simulink model "Filter_main"  (R2023a)
settings: Solver=FixedStepDiscrete  StartTime=0.0  StopTime=2  FixedStep=Ts  RelTol=1e-3
InitFcn:
  | Ts=5e-6;
  | f=50;
  | w=2*pi*f;
libraries: spsThreePhaseSeriesRLCBranchLib x7, spsGroundLib x5, spsSeriesRLCBranchLib x3, spsThreePhaseVIMeasurementLib x3, powerlib_extras x2, spsRMSLib x2, spsTHDLib x2, spsThreePhaseParallelRLCLoadLib x2, spsThreePhaseHarmonicFilterLib x1, dspxfrm3 x1, spsPower3phInstantaneousLib x1, spsThreePhaseBreakerLib x1
settings Model: Creator=Aminsystem  LastModifiedBy=Aminsystem
settings DataIOCC: SaveOutput=off  SignalLogging=off  DSMLogging=off  SaveTime=off  ReturnWorkspaceOutputs=off

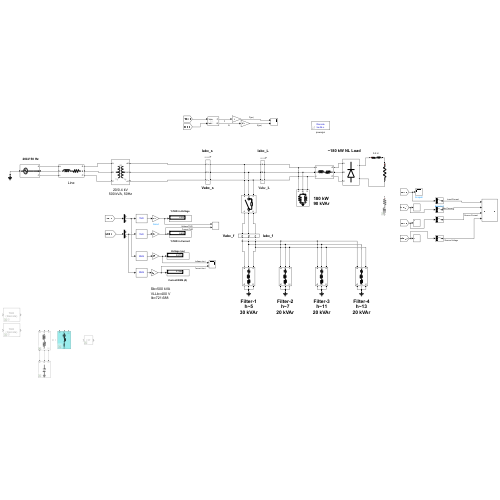
[thumbnail: Simulink's stored preview of the top-level diagram]
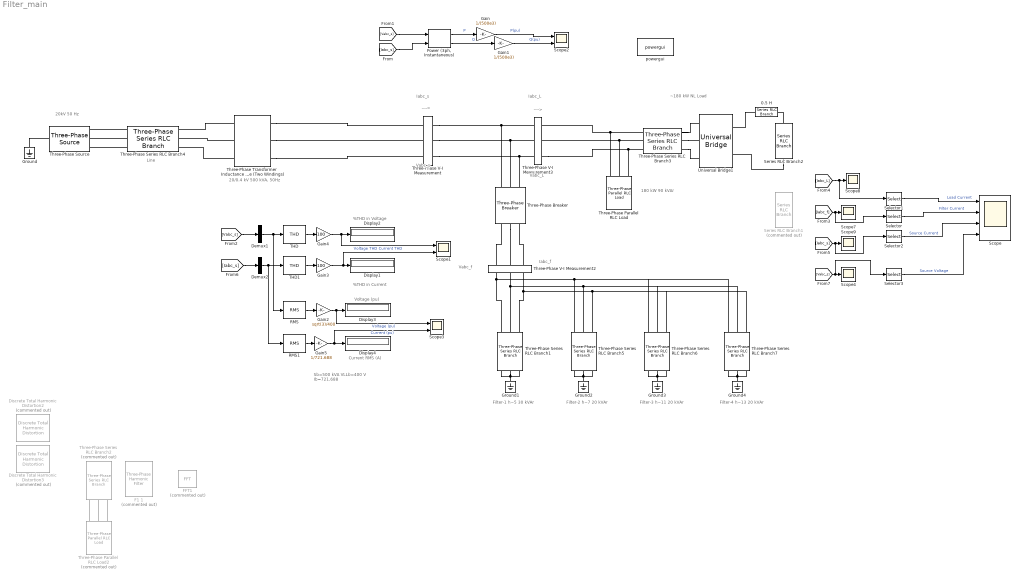
== system Filter_main ==
  note: Sb=500 kVA
      | VLLb=400 V
      | Ib=721.688
  note: %THD in Current
  note: %THD in Voltage
  note: ~180 kW NL Load
  note: Line
  note: Filter-1
      | h~5
      | 30 kVAr
  note: 180 kW
      | 90 kVAr
  note: 20kV 50 Hz
  note: Iabc_L
  note: Vabc_s
  note: Iabc_s
  note: ---->
  note: ---->
  note: Vabc_L
  note: Iabc_f
  note: Vabc_f
  note: 20/0.4 kV
      | 500 kVA, 50Hz
  note: Filter-2
      | h~7
      | 20 kVAr
  note: Filter-3
      | h~11
      | 20 kVAr
  note: Filter-4
      | h~13
      | 20 kVAr
  note: Voltage (pu)
  note: Current RMS (A)
  "0.5 H " : spsSeriesRLCBranchLib/Series RLC Branch  LConnTagsString=__new0  RConnTagsString=__new0  BranchType=RL  Resistance=0.5  Inductance=1e-3  SetiL0=off  InitialCurrent=0  Capacitance=1.0  Setx0=off  InitialVoltage=0  Measurements=None
  Demux1 : Demux  Outputs=3
  Demux2 : Demux  Outputs=3
  Discrete Total Harmonic Distortion2 : powerlib_extras/Discrete Measurements/Discrete Total Harmonic Distortion  Commented=on  Freq=50  Ts=50e-6
  Discrete Total Harmonic Distortion3 : powerlib_extras/Discrete Measurements/Discrete Total Harmonic Distortion  Commented=on  Freq=50  Ts=50e-6
  Display{1..4} (4 alike) : Display
  F1 1 : spsThreePhaseHarmonicFilterLib/Three-Phase Harmonic Filter  Commented=on  LConnTagsString=A|B|C  FilterType=Single-tuned  FilterConnection=Y (grounded)  ParNom=[400 50]  Qc=30e3  Fr=[5*50]  Frd=[11*60 13*60]  Q=5  Measurements=None
      settings: AttributesFormatString=\n
  FFT1 : dspxfrm3/FFT  Commented=on  FFTImplementation=Auto  CompMethod=Table lookup  TableOpt=NEW  TableOptActive=Speed  BitRevOrder=off  Normalize=off  InheritFFTLength=on  FFTLength=64  WrapInput=on  roundingMode=Floor  overflowMode=off  firstCoeffDataTypeStr=Inherit: Same word length as input  firstCoeffLastDataTypeStr=Inherit: Same word length as input  outputMin=[]  outputMax=[]
  Gain : Gain  Gain=1/(500e3)
  Gain1 : Gain  Gain=1/(500e3)
  Gain2 : Gain  Gain=sqrt(3)/400
  Gain3 : Gain  Gain=100
  Gain4 : Gain  Gain=100
  Gain5 : Gain  Gain=1/721.688
  Ground{,1..4} (5 alike) : spsGroundLib/Ground  LConnTagsString=a
  "Power (3ph, Instantaneous)" : spsPower3phInstantaneousLib/Power (3ph, Instantaneous)
  RMS : spsRMSLib/RMS  TrueRMS=on  Freq=50  RMSInit=230  Ts=Ts
  RMS1 : spsRMSLib/RMS  TrueRMS=on  Freq=50  RMSInit=0  Ts=Ts
  Scope : Scope  NumInputPorts=4
  Scope1 : Scope  NumInputPorts=2
  Scope2 : Scope  NumInputPorts=2
  Scope3 : Scope  NumInputPorts=2
  Scope{4,7..9} (4 alike) : Scope
  Selector{,1..3} (4 alike) : Selector  InputPortWidth=3  IndexOptions=Index vector (dialog)  Indices=[1]  OutputSizes=1
  Series RLC Branch1 : spsSeriesRLCBranchLib/Series RLC Branch  Commented=on  LConnTagsString=__new0  RConnTagsString=__new0  BranchType=RL  Resistance=2  Inductance=0.5e-3  SetiL0=off  InitialCurrent=0  Capacitance=1e-6  Setx0=off  InitialVoltage=0  Measurements=None
  Series RLC Branch2 : spsSeriesRLCBranchLib/Series RLC Branch  LConnTagsString=__new0  RConnTagsString=__new0  BranchType=R  Resistance=400*400/180e3  Inductance=0.5e-3  SetiL0=off  InitialCurrent=0  Capacitance=1e-6  Setx0=off  InitialVoltage=0  Measurements=None
  THD : spsTHDLib/THD  Freq=50  Ts=Ts
  THD1 : spsTHDLib/THD  Freq=50  Ts=Ts
  Three-Phase Parallel RLC Load : spsThreePhaseParallelRLCLoadLib/Three-Phase Parallel RLC Load  LConnTagsString=A|B|C  Configuration=Y (grounded)  NominalVoltage=400  Vabc=[1e3 1e3 1e3]  Vabcp=[1e3 1e3 1e3]  NominalFrequency=50  UnbalancedPower=off  ActivePower=180e3  InductivePower=90e3  CapacitivePower=0  Pabc=[10e3 9e3 11e3]  QLabc=[100 90 110]  QCabc=[100 90 110]  Pabcp=[10e3 9e3 11e3]  QLabcp=[100 90 110]  QCabcp=[100 90 110]  Measurements=None  LoadType=constant Z
  Three-Phase Parallel RLC Load2 : spsThreePhaseParallelRLCLoadLib/Three-Phase Parallel RLC Load  Commented=on  LConnTagsString=A|B|C  Configuration=Y (grounded)  NominalVoltage=400  Vabc=[1e3 1e3 1e3]  Vabcp=[1e3 1e3 1e3]  NominalFrequency=50  UnbalancedPower=off  ActivePower=0  InductivePower=0  CapacitivePower=90e3  Pabc=[10e3 9e3 11e3]  QLabc=[100 90 110]  QCabc=[100 90 110]  Pabcp=[10e3 9e3 11e3]  QLabcp=[100 90 110]  QCabcp=[100 90 110]  Measurements=None  LoadType=constant Z
  Three-Phase Series RLC Branch1 : spsThreePhaseSeriesRLCBranchLib/Three-Phase Series RLC Branch  LConnTagsString=A|B|C  RConnTagsString=A|B|C  BranchType=RLC  Resistance=1.142/100  Inductance=0.779e-3  Capacitance=30e3/(400*400*w)  Measurements=None
  Three-Phase Series RLC Branch2 : spsThreePhaseSeriesRLCBranchLib/Three-Phase Series RLC Branch  Commented=on  LConnTagsString=A|B|C  RConnTagsString=A|B|C  BranchType=RL  Resistance=1e-3  Inductance=0.1e-3  Capacitance=1e-6  Measurements=None
  Three-Phase Series RLC Branch3 : spsThreePhaseSeriesRLCBranchLib/Three-Phase Series RLC Branch  LConnTagsString=A|B|C  RConnTagsString=A|B|C  BranchType=RL  Resistance=0.1e-3  Inductance=0.1e-3  Capacitance=1e-6  Measurements=None
  Three-Phase Series RLC Branch4 : spsThreePhaseSeriesRLCBranchLib/Three-Phase Series RLC Branch  LConnTagsString=A|B|C  RConnTagsString=A|B|C  BranchType=RL  Resistance=1  Inductance=16e-3  Capacitance=1e-6  Measurements=None
  Three-Phase Series RLC Branch5 : spsThreePhaseSeriesRLCBranchLib/Three-Phase Series RLC Branch  LConnTagsString=A|B|C  RConnTagsString=A|B|C  BranchType=RLC  Resistance=1.210/100  Inductance=0.583e-3  Capacitance=20e3/(400*400*w)  Measurements=None
  Three-Phase Series RLC Branch6 : spsThreePhaseSeriesRLCBranchLib/Three-Phase Series RLC Branch  LConnTagsString=A|B|C  RConnTagsString=A|B|C  BranchType=RLC  Resistance=0.765/100  Inductance=0.233e-3  Capacitance=20e3/(400*400*w)  Measurements=None
  Three-Phase Series RLC Branch7 : spsThreePhaseSeriesRLCBranchLib/Three-Phase Series RLC Branch  LConnTagsString=A|B|C  RConnTagsString=A|B|C  BranchType=RLC  Resistance=0.646/100  Inductance=0.166e-3  Capacitance=20e3/(400*400*w)  Measurements=None
  Three-Phase V-I Measurement : spsThreePhaseVIMeasurementLib/Three-Phase V-I Measurement  VoltageMeasurement=phase-to-ground  SetLabelV=on  LabelV=Vabc_s  Vpu=off  VpuLL=off  CurrentMeasurement=yes  SetLabelI=on  LabelI=Iabc_s  Ipu=off  Pbase=100e6  Vbase=500e3  OutputType=Complex  PhasorSimulation=off  PSBequivalent=0
  Three-Phase V-I Measurement2 : spsThreePhaseVIMeasurementLib/Three-Phase V-I Measurement  VoltageMeasurement=phase-to-ground  SetLabelV=on  LabelV=Vabc_f  Vpu=off  VpuLL=off  CurrentMeasurement=yes  SetLabelI=on  LabelI=Iabc_f  Ipu=off  Pbase=100e6  Vbase=500e3  OutputType=Complex  PhasorSimulation=off  PSBequivalent=0
  Three-Phase V-I Measurement3 : spsThreePhaseVIMeasurementLib/Three-Phase V-I Measurement  VoltageMeasurement=phase-to-ground  SetLabelV=on  LabelV=Vabc_L  Vpu=off  VpuLL=off  CurrentMeasurement=yes  SetLabelI=on  LabelI=Iabc_L  Ipu=off  Pbase=100e6  Vbase=500e3  OutputType=Complex  PhasorSimulation=off  PSBequivalent=0
  Three-Phase Breaker : spsThreePhaseBreakerLib/Three-Phase Breaker  InitialState=open  SwitchA=on  SwitchB=on  SwitchC=on  SwitchTimes=[1]  External=off  BreakerResistance=0.001  SnubberResistance=1e7  SnubberCapacitance=inf  Measurements=None
  Three-Phase Source : spsThreePhaseSourceLib/Three-Phase Source  InternalConnection=Yn  VoltagePhases=off  Voltage=20e3  PhaseAngle=0  Voltage_phases=[25e3 25e3 25e3]/sqrt(3)  PhaseAngles_phases=[0 -120 +120]  Frequency=50  NonIdealSource=off  SpecifyImpedance=off  Resistance=0.8929  Inductance=16.58e-3  ShortCircuitLevel=100e6  BaseVoltage=20e3  XRratio=10  BusType=swing  Pref=10e3  Qref=0  Prefabc=[10e3, 10e3, 10e3]  Qrefabc=[0, 0, 0]  Qmin=-inf  Qmax=inf
  Three-Phase Transformer Inductance Matrix Type (Two Windings) : spsThreePhaseTransformerInductanceMatrixTypeTwoWindingsLib/Three-Phase Transformer Inductance Matrix Type (Two Windings)  CoreType=Three single-phase cores  Winding1Connection=Yg  Winding2Connection=Yg  AutoTransformer=off  Measurements=None  NominalPower=[500e3, 50]  VLLnom=[20e3, 400]  WindingResistances=[0.01, 0.01]  NoLoadIexcPos=2  NoLoadPlossPos=250  ShortCircuitReactancePos=0.06  ShortCircuitReactancePosAuto=0.06  NoLoadIexcZero=100  NoLoadPlossZero=1500  ShortCircuitReactanceZero=0.03  ShortCircuitReactanceZeroAuto=0.03
      settings: LibrarySourceBlock=|
      | sps_lib/Power Grid Elements/Three-Phase Transformer
      | Inductance Matrix Type
      | (Two Windings)
  Universal Bridge1 : spsUniversalBridgeLib/Universal Bridge  Arms=3  SnubberResistance=1e5  SnubberCapacitance=inf  Device=Diodes  Ron=1e-3  Lon=0  ForwardVoltages="[  0  0  ]"  ForwardVoltage=0  GTOparameters=[ 10e-6 , 20e-6 ]  IGBTparameters=[ 1e-6 , 2e-6 ]  Measurements=None  Measurements_2=None  converterType=Rectifier
  powergui : sps_lib/powergui  Priority=1  SimulationMode=Discrete  SampleTime=Ts  frequency=60  Iterations=50  frequencyindice=50  Pbase=100e6  ErrMax=1e-4  UnitsV=kV  UnitsW=MW  buscounter=0  FunctionMessages=off  echomessages=off  EnableUseOfTLC=off  CurrentSourceSwitches=off  DisableSnubberDevices=off  DisableRonSwitches=off  DisableVfSwitches=off  DisplayEquations=off  AutomaticDiscreteSolvers=off  SolverType=Tustin  Interpol=off  ExternalGateDelay=off  methode=off  Ts=100  x0status=blocks  SPID=on  SwTol=0  HookPort=off  NonlinearTolerance=1e-4  nMaxIteration=100  ContinueOnMaxIteration=off  RestoreLinks=warning  ResistiveCurrentMeasurement=off  Frange=[0:2:500]  Ylog=off  Xlog=on  ShowGrid=off  save=off  variable=ZData  structure=Iabc_s  ZoomFFT=off  StartTime=1.6  cycles=20  DisplayStyle=1  fundamental=50  FreqAxis=on  MaxFrequency=50*20  frequencyindicesteady=1  RmsSteady=1  display=off
  wires:
  [Iabc_L] -> Selector1/1, Scope8/1
  [Iabc_s] -> Selector2/1, Scope9/1
  [Iabc_f] -> Selector/1, Scope7/1
  Selector1/1 -> Scope/1  "Load Current"
  Selector/1 -> Scope/2  "Filter Current"
  Selector2/1 -> Scope/3  "Source Current"
  [Vabc_s] -> "Power (3ph, Instantaneous)"/1
  [Iabc_s] -> "Power (3ph, Instantaneous)"/2
  "Power (3ph, Instantaneous)"/1 -> Gain/1  "P"
  "Power (3ph, Instantaneous)"/2 -> Gain1/1  "Q"
  Gain/1 -> Scope2/1  "P(pu)"
  Gain1/1 -> Scope2/2  "Q(pu)"
  [Iabc_s] -> Demux2/1
  Demux2/2 -> RMS1/1, THD1/1
  Demux1/2 -> RMS/1, THD/1
  [Vabc_s] -> Demux1/1
  Gain3/1 -> Scope1/2, Display1/1  "Current THD"
  THD1/1 -> Gain3/1
  THD/1 -> Gain4/1
  Gain4/1 -> Scope1/1, Display2/1  "Voltage THD"
  RMS/1 -> Gain2/1
  RMS1/1 -> Gain5/1
  Gain2/1 -> Scope3/1, Display3/1  "Voltage (pu)"
  Gain5/1 -> Scope3/2, Display4/1  "Current (pu)"
  [Vabc_s] -> Selector3/1, Scope4/1
  Selector3/1 -> Scope/4  "Source Voltage"
  connections:
  Three-Phase Series RLC Branch3/RConn2 -- Three-Phase V-I Measurement3/RConn2 -- Three-Phase Parallel RLC Load/LConn2
  Three-Phase V-I Measurement2/RConn1 -- Three-Phase Breaker/LConn1
  Three-Phase V-I Measurement3/RConn3 -- Three-Phase Parallel RLC Load/LConn3 -- Three-Phase Series RLC Branch3/RConn3
  Three-Phase Series RLC Branch3/RConn1 -- Three-Phase V-I Measurement3/RConn1 -- Three-Phase Parallel RLC Load/LConn1
  Series RLC Branch2/RConn1 -- Universal Bridge1/RConn2
  Series RLC Branch2/LConn1 -- "0.5 H "/RConn1
  Three-Phase Series RLC Branch3/LConn2 -- Universal Bridge1/LConn2
  Three-Phase Series RLC Branch3/LConn1 -- Universal Bridge1/LConn1
  Three-Phase Series RLC Branch3/LConn3 -- Universal Bridge1/LConn3
  Three-Phase Breaker/LConn2 -- Three-Phase V-I Measurement2/RConn2
  Three-Phase V-I Measurement/RConn3 -- Three-Phase Breaker/RConn3 -- Three-Phase V-I Measurement3/LConn3
  Ground/LConn1 -- Three-Phase Source/LConn1
  Three-Phase V-I Measurement2/RConn3 -- Three-Phase Breaker/LConn3
  Three-Phase V-I Measurement/RConn1 -- Three-Phase Breaker/RConn1 -- Three-Phase V-I Measurement3/LConn1
  Three-Phase V-I Measurement/RConn2 -- Three-Phase Breaker/RConn2 -- Three-Phase V-I Measurement3/LConn2
  Three-Phase Parallel RLC Load2/LConn3 -- Three-Phase Series RLC Branch2/LConn3
  Three-Phase Parallel RLC Load2/LConn2 -- Three-Phase Series RLC Branch2/LConn2
  Three-Phase Parallel RLC Load2/LConn1 -- Three-Phase Series RLC Branch2/LConn1
  Three-Phase Series RLC Branch1/LConn1 -- Ground1/LConn1 -- Three-Phase Series RLC Branch1/LConn2 -- Three-Phase Series RLC Branch1/LConn3
  Three-Phase Series RLC Branch1/RConn2 -- Three-Phase Series RLC Branch7/RConn2 -- Three-Phase Series RLC Branch6/RConn2 -- Three-Phase Series RLC Branch5/RConn2 -- Three-Phase V-I Measurement2/LConn2
  Three-Phase Series RLC Branch1/RConn1 -- Three-Phase Series RLC Branch7/RConn1 -- Three-Phase Series RLC Branch6/RConn1 -- Three-Phase Series RLC Branch5/RConn1 -- Three-Phase V-I Measurement2/LConn1
  Three-Phase Series RLC Branch1/RConn3 -- Three-Phase Series RLC Branch7/RConn3 -- Three-Phase Series RLC Branch6/RConn3 -- Three-Phase Series RLC Branch5/RConn3 -- Three-Phase V-I Measurement2/LConn3
  "0.5 H "/LConn1 -- Universal Bridge1/RConn1
  Three-Phase Series RLC Branch4/RConn1 -- Three-Phase Source/RConn1
  Three-Phase Series RLC Branch4/RConn3 -- Three-Phase Source/RConn3
  Three-Phase Series RLC Branch4/RConn2 -- Three-Phase Source/RConn2
  Three-Phase Transformer Inductance Matrix Type (Two Windings)/LConn2 -- Three-Phase Series RLC Branch4/LConn2
  Three-Phase Transformer Inductance Matrix Type (Two Windings)/LConn1 -- Three-Phase Series RLC Branch4/LConn1
  Three-Phase Transformer Inductance Matrix Type (Two Windings)/LConn3 -- Three-Phase Series RLC Branch4/LConn3
  Ground2/LConn1 -- Three-Phase Series RLC Branch5/LConn1 -- Three-Phase Series RLC Branch5/LConn3 -- Three-Phase Series RLC Branch5/LConn2
  Three-Phase Series RLC Branch6/LConn1 -- Ground3/LConn1 -- Three-Phase Series RLC Branch6/LConn2 -- Three-Phase Series RLC Branch6/LConn3
  Ground4/LConn1 -- Three-Phase Series RLC Branch7/LConn1 -- Three-Phase Series RLC Branch7/LConn3 -- Three-Phase Series RLC Branch7/LConn2
  Three-Phase Transformer Inductance Matrix Type (Two Windings)/RConn1 -- Three-Phase V-I Measurement/LConn1
  Three-Phase Transformer Inductance Matrix Type (Two Windings)/RConn2 -- Three-Phase V-I Measurement/LConn2
  Three-Phase Transformer Inductance Matrix Type (Two Windings)/RConn3 -- Three-Phase V-I Measurement/LConn3
